simulink library "arsenal"  (R2025b)
settings: Solver=VariableStepAuto  StartTime=0.0  StopTime=10.0  RelTol=1e-3
undefined symbols (not defined in the file or in its folder): DiscIntNeverNeededParam, Kd
libraries: fl_lib x21, sdl_lib x4, simulink x3, dspstat3 x2, ee_lib x2, nesl_utility x2, simulink_extras x1, slpidlib x1
settings Model: Creator=upattacini  LastModifiedBy=upattacini

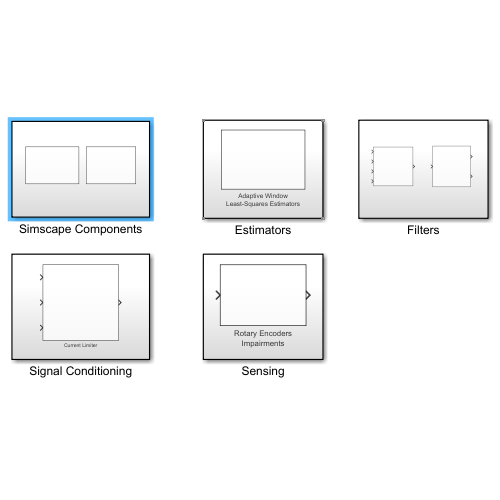
[thumbnail: Simulink's stored preview of the top-level diagram]
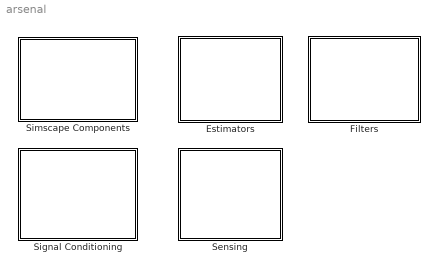
== system arsenal ==
  Estimators : Subsystem
  Filters : Subsystem
  Sensing : Subsystem
  Signal Conditioning : Subsystem
  Simscape Components : Subsystem

== system arsenal/Estimators ==
  Adaptive Window Least-Squares Estimators : Subsystem

== system arsenal/Filters ==
  Adaptive Exponential Smoother : Subsystem  mask(Exponential Adaptive Smoother){eta=0, m=0, V0=0}
      mask prompts: eta "Learning rate"; m "Momentum rate"; V0 "Initial variance estimate"
      mask help: Smooths out a noisy signal by estimating its variance at each time step. Use the learning rate to adjust the convergence speed and the momentum rate to weigh the noise applied to the gradient.
      mask Display:
      | port_label('input', 1, 'x','texmode', 'on');
      | port_label('output', 1, 'y','texmode', 'on');
      | port_label('output', 2, '\sigma^2_{est}','texmode', 'on');
  Discrete Minimum Jerk : Subsystem  mask(Minimum Jerk Filter){Ts=0.001}
      mask prompts: Ts "Sample time (s)"
      mask help:
      | Apply quasi-minimum jerk filtering to the input.
      | The filter reactivity can be adjusted via the input T, which specifies the rise-time.
      | The filter can be reset to output the initial value out0.

== system arsenal/Sensing ==
  Rotary Encoders Impairments : Subsystem  mask(Rotary Encoders Impairments){bit_resolution=14, bit_noise=2, seed=0, Ts=0.001}
      mask prompts: bit_resolution "Bits or resolution"; bit_noise "Bits of noise"; Ts "Sample time (s)"
      mask help:
      | Simulate the impairments underlying the rotary encoders readouts.
      | In particular, the block simulates the effects of quantization and noise.

== system arsenal/Signal Conditioning ==
  Current Limiter : Subsystem  mask(Current Limiter){Ts=0.00005, I_max_gain=0.1, Discrete_time_integrator_gain=1.0}
      mask prompts: Ts "Sample Time (s):"; I_max_gain "I Max Gain:"; Discrete_time_integrator_gain "Discrete-Time Integrator Gain:"
      mask help: This block limits the magnitude of an input current signal to a specified maximum value, preventing it from exceeding safe operating boundaries. It acts as a saturation filter to protect downstream components (such as motor drivers or actuators) from overcurrent conditions.
      mask TypeOptions Ts:
      | Discrete-Time
      | Integrator/SampleTime | Unit Delay/SampleTime
      mask TypeOptions I_max_gain: I_max_gain/Gain
      mask TypeOptions Discrete_time_integrator_gain:
      | Discrete-Time
      | Integrator/gainval

== system arsenal/Simscape Components ==
  Actuators : Subsystem
  Transmissions : Subsystem

== system arsenal/Estimators/Adaptive Window Least-Squares Estimators ==
  AWLS Estimator 1st-order : MATLAB Function  Description=This block implements adaptive window techniques as per https://dx.doi.org/10.1109/87.880606.  TreatAsAtomicUnit=on
  AWLS Estimator 2nd-order : MATLAB Function  Description=This block implements adaptive window techniques as per https://dx.doi.org/10.1109/87.880606.  TreatAsAtomicUnit=on

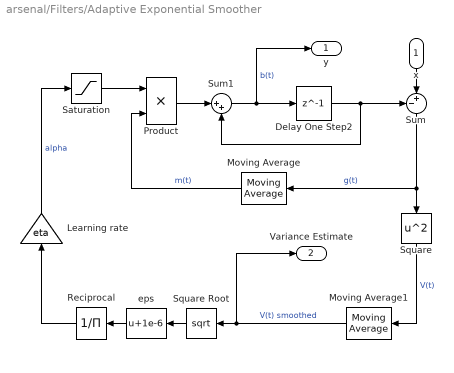
== system arsenal/Filters/Adaptive Exponential Smoother ==
  x : Inport  OutDataTypeStr=single
  Delay One Step2 : Delay  DelayLength=1  InitialCondition=0
  Learning rate : Gain  Gain=eta
  Moving Average : dspstat3/Moving Average  Method=Exponential weighting  ForgettingFactorPort=off  SpecifyWindowLength=on  WindowLength=4  OverlapLength=3  AllowArbitraryInputLength=off  ForgettingFactor=m  SimulateUsing=Code generation
  Moving Average1 : dspstat3/Moving Average  Method=Exponential weighting  ForgettingFactorPort=off  SpecifyWindowLength=on  WindowLength=4  OverlapLength=3  AllowArbitraryInputLength=off  ForgettingFactor=m  SimulateUsing=Code generation
  Product : Product
  Reciprocal : Product  Inputs=/  CollapseDim=2
  Saturation : Saturate  UpperLimit=0.99999  LowerLimit=1e-6
  Square : Math  Operator=square
  Square Root : Sqrt
  Sum : Sum  Inputs=-+|
  Sum1 : Sum  Inputs=|++
  eps : Bias  Bias=1e-6  SaturateOnIntegerOverflow=off
  y : Outport  OutDataTypeStr=single
  Variance Estimate : Outport  Port=2  VectorParamsAs1DForOutWhenUnconnected=off
  wires:
  Square Root/1 -> eps/1
  Sum/1 -> Moving Average/1, Square/1  "g(t)"
  eps/1 -> Reciprocal/1
  x/1 -> Sum/2
  Saturation/1 -> Product/1
  Reciprocal/1 -> Learning rate/1
  Learning rate/1 -> Saturation/1  "alpha"
  Product/1 -> Sum1/1
  Moving Average/1 -> Product/2  "m(t)"
  Moving Average1/1 -> Variance Estimate/1, Square Root/1  "V(t) smoothed"
  Square/1 -> Moving Average1/1  "V(t)"
  Sum1/1 -> Delay One Step2/1, y/1  "b(t)"
  Delay One Step2/1 -> Sum1/2, Sum/1

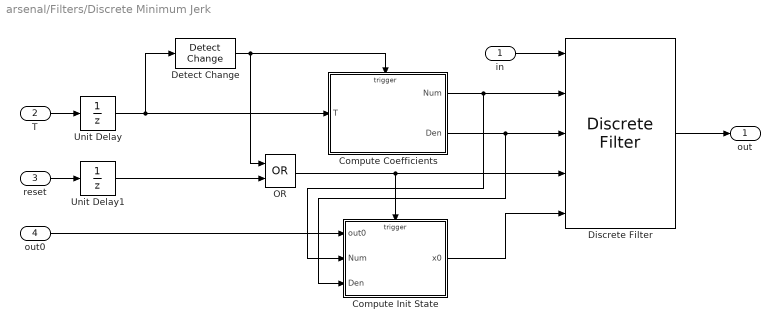
== system arsenal/Filters/Discrete Minimum Jerk ==
  in : Inport  PortDimensions=1
  T : Inport  Port=2  PortDimensions=1
  reset : Inport  Port=3  PortDimensions=1
  out0 : Inport  Port=4  PortDimensions=1
  Compute Coefficients : Subsystem
  Compute Init State : Subsystem  TreatAsAtomicUnit=on
  Detect Change : simulink/Logic and Bit Operations/Detect Change  vinit=0  OutDataTypeStr=uint8
  Discrete Filter : DiscreteFilter  NumeratorSource=Input port  DenominatorSource=Input port  InitialStatesSource=Input port  ExternalReset=Rising  a0EqualsOne=on
      settings: InputPortMap=u0,p1,p3,r7,p5
  OR : Logic  Operator=OR  AllPortsSameDT=off  OutDataTypeStr=boolean
  Unit Delay : UnitDelay  SampleTime=-1  HasFrameUpgradeWarning=on
  Unit Delay1 : UnitDelay  SampleTime=-1  HasFrameUpgradeWarning=on
  out : Outport  PortDimensions=1
  wires:
  in/1 -> Discrete Filter/1
  Discrete Filter/1 -> out/1
  T/1 -> Unit Delay/1
  Detect Change/1 -> Compute Coefficients/Trigger, OR/1
  Compute Coefficients/1(Num) -> Compute Init State/2(Num), Discrete Filter/2
  Compute Coefficients/2(Den) -> Compute Init State/3(Den), Discrete Filter/3
  Unit Delay/1 -> Compute Coefficients/1(T), Detect Change/1
  reset/1 -> Unit Delay1/1
  out0/1 -> Compute Init State/1(out0)
  Compute Init State/1(x0) -> Discrete Filter/5
  Unit Delay1/1 -> OR/2
  OR/1 -> Compute Init State/Trigger, Discrete Filter/4

== system arsenal/Sensing/Rotary Encoders Impairments ==
  in : Inport
  Quantization and Noise : Subsystem  mask{bit_resolution=bit_resolution, bit_noise=bit_noise, seed=0, Ts=Ts}
      mask prompts: bit_resolution "Resolution bits"; bit_noise "Noise bits"; Ts "Sample time (s)"
      settings: PortSchema="{\"entries\":[{\"content\":{\"sides\":[{\"content\":{\"connectorIds\":[\"Out1\"]},\"type\":\"ConnectorPlacement.EquallySpacedRectSide\",\"uuid\":\"5c60203e-1477-4c63-bf85-2a9264896243\"},{\"content\":{\"connectorIds\":[\"In1\"],\"side\":\"RIGHT\"},\"type\":\"ConnectorPlacement.EquallySpacedRectSide\",\"uuid\":\"fde9215e-0eee-4b90-b3d3-bc5e0578faf0\"},{\"content\":{\"side\":\"TOP\"},\"type\":\"ConnectorPlacement.EquallySpacedRectSide\",\"uuid\":\"75472767-9856-4b99-a0f4-bd856ef58e73\"}]},\"type\":\"ConnectorPlacement.EquallySpacedConnector\",\"uuid\":\"089ac2bf-9317-43ab-ab34-2d9e1bbbe948\"}],\"packageUris\":[\"http://schema.mathworks.com/mf0/Connector/R2020b\"],\"version\":\"1.0\"}"
  Signal Specification : SignalSpecification  Unit=deg
  Signal Specification1 : SignalSpecification  Unit=deg
  out : Outport
  wires:
  in/1 -> Signal Specification1/1
  Quantization and Noise/1(out) -> Signal Specification/1
  Signal Specification/1 -> out/1
  Signal Specification1/1 -> Quantization and Noise/1(in)

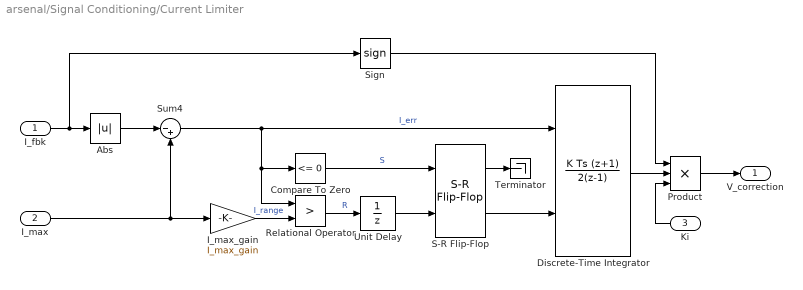
== system arsenal/Signal Conditioning/Current Limiter ==
  I_fbk : Inport
  I_max : Inport  Port=2
  Ki : Inport  Port=3
  Abs : Abs  ZeroCross=off  SaturateOnIntegerOverflow=off
  Compare To Zero : simulink/Logic and Bit Operations/Compare To Zero  relop=<=  OutDataTypeStr=boolean
  Discrete-Time Integrator : DiscreteIntegrator  IntegratorMethod=Integration: Trapezoidal  gainval=Discrete_time_integrator_gain  ExternalReset=level  SampleTime=Ts  ICPrevOutput=DiscIntNeverNeededParam  ICPrevScaledInput=DiscIntNeverNeededParam
  I_max_gain : Gain  Gain=I_max_gain  OutDataTypeStr=single
  Product : Product  Inputs=3
  Relational Operator : RelationalOperator  Operator=>  OutDataTypeStr=boolean  RndMeth=Simplest  InputSameDT=off
  S-R Flip-Flop : simulink_extras/Flip Flops/S-R Flip-Flop  initial_condition=0
  Sign : Signum
  Sum4 : Sum  Inputs=|-+
  Terminator : Terminator
  Unit Delay : UnitDelay  SampleTime=Ts  HasFrameUpgradeWarning=on
  V_correction : Outport
  wires:
  Discrete-Time Integrator/1 -> Product/2
  I_max_gain/1 -> Relational Operator/2  "I_range"
  S-R Flip-Flop/1 -> Terminator/1
  Abs/1 -> Sum4/1
  Sign/1 -> Product/1
  S-R Flip-Flop/2 -> Discrete-Time Integrator/2
  Sum4/1 -> Relational Operator/1, Compare To Zero/1, Discrete-Time Integrator/1  "I_err"
  Ki/1 -> Product/3
  I_fbk/1 -> Sign/1, Abs/1
  Compare To Zero/1 -> S-R Flip-Flop/1  "S"
  Relational Operator/1 -> Unit Delay/1  "R"
  I_max/1 -> Sum4/2, I_max_gain/1
  Product/1 -> V_correction/1
  Unit Delay/1 -> S-R Flip-Flop/2

== system arsenal/Simscape Components/Actuators ==
  DC Motors : Subsystem

== system arsenal/Simscape Components/Transmissions ==
  Harmonic Drives : Subsystem

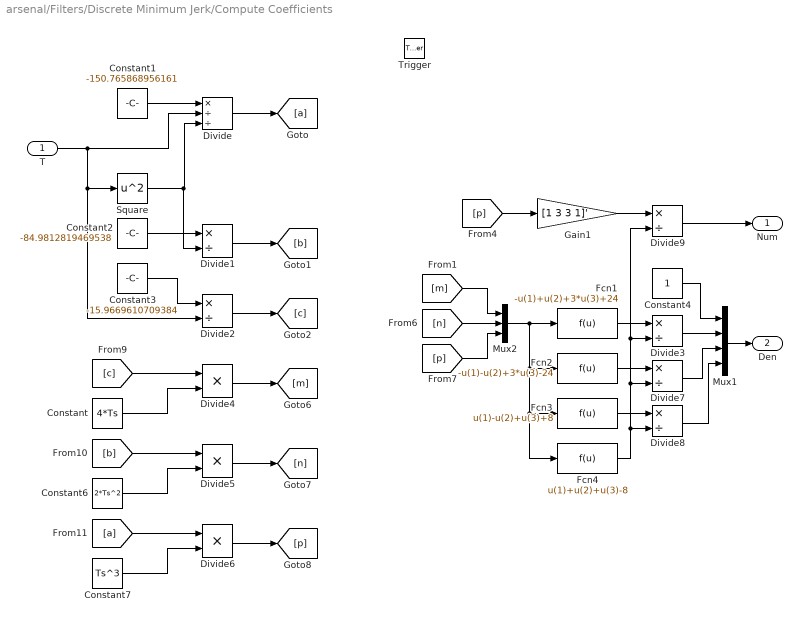
== system arsenal/Filters/Discrete Minimum Jerk/Compute Coefficients ==
  T : Inport
  Trigger : TriggerPort  VariantControl=(inherit)  PortDimensions=1
  Constant : Constant  Value=4*Ts
  Constant1 : Constant  Value=-150.765868956161
  Constant2 : Constant  Value=-84.9812819469538
  Constant3 : Constant  Value=-15.9669610709384
  Constant4 : Constant
  Constant6 : Constant  Value=2*Ts^2
  Constant7 : Constant  Value=Ts^3
  Divide : Product  Inputs=*//
  Divide{1..3,7..9} (6 alike) : Product  Inputs=*/
  Divide4 : Product  Inputs=**
  Divide5 : Product  Inputs=**
  Divide6 : Product  Inputs=**
  Fcn1 : Fcn  Expr=-u(1)+u(2)+3*u(3)+24
  Fcn2 : Fcn  Expr=-u(1)-u(2)+3*u(3)-24
  Fcn3 : Fcn  Expr=u(1)-u(2)+u(3)+8
  Fcn4 : Fcn  Expr=u(1)+u(2)+u(3)-8
  Gain1 : Gain  Gain=[1 3 3 1]'
  Mux1 : Mux
  Mux2 : Mux  Inputs=3
  Square : Math  Operator=square
  Num : Outport  InitialOutput=[0 0 0 0]
  Den : Outport  Port=2  InitialOutput=[1 0 0 0]'
  wires:
  Divide9/1 -> Num/1
  Gain1/1 -> Divide9/1
  Fcn4/1 -> Divide3/2, Divide9/2, Divide7/2, Divide8/2
  Fcn3/1 -> Divide8/1
  Fcn2/1 -> Divide7/1
  Divide8/1 -> Mux1/4
  Divide7/1 -> Mux1/3
  Divide3/1 -> Mux1/2
  Fcn1/1 -> Divide3/1
  Mux2/1 -> Fcn1/1, Fcn2/1, Fcn3/1, Fcn4/1
  [p] -> Mux2/3
  [n] -> Mux2/2
  [m] -> Mux2/1
  Constant7/1 -> Divide6/2
  [a] -> Divide6/1
  Divide6/1 -> [p]
  Divide5/1 -> [n]
  [b] -> Divide5/1
  Constant6/1 -> Divide5/2
  Constant/1 -> Divide4/2
  [c] -> Divide4/1
  Divide4/1 -> [m]
  Mux1/1 -> Den/1
  Constant4/1 -> Mux1/1
  Divide/1 -> [a]
  Square/1 -> Divide/3, Divide1/2
  Constant3/1 -> Divide2/1
  Constant2/1 -> Divide1/1
  [p] -> Gain1/1
  Divide2/1 -> [c]
  T/1 -> Divide/2, Square/1, Divide2/2
  Divide1/1 -> [b]
  Constant1/1 -> Divide/1

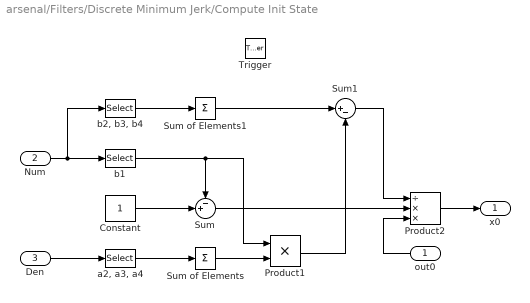
== system arsenal/Filters/Discrete Minimum Jerk/Compute Init State ==
  out0 : Inport
  Num : Inport  Port=2
  Den : Inport  Port=3
  Trigger : TriggerPort  VariantControl=(inherit)
  Constant : Constant
  Product1 : Product
  Product2 : Product  Inputs=/**
  Sum : Sum  Inputs=-+|
  Sum of Elements : Sum  Inputs=+
  Sum of Elements1 : Sum  Inputs=+
  Sum1 : Sum  Inputs=|+-
  "a2, a3, a4" : Selector  InputPortWidth=4  IndexOptions=Index vector (dialog)  Indices=[2 3 4]  OutputSizes=1
  b1 : Selector  InputPortWidth=4  IndexOptions=Index vector (dialog)  Indices=1  OutputSizes=1
  "b2, b3, b4" : Selector  InputPortWidth=4  IndexOptions=Index vector (dialog)  Indices=[2 3 4]  OutputSizes=1
  x0 : Outport
  wires:
  Den/1 -> "a2, a3, a4"/1
  Num/1 -> "b2, b3, b4"/1, b1/1
  Constant/1 -> Sum/2
  b1/1 -> Sum/1, Product1/1
  "a2, a3, a4"/1 -> Sum of Elements/1
  "b2, b3, b4"/1 -> Sum of Elements1/1
  Sum of Elements/1 -> Product1/2
  Sum of Elements1/1 -> Sum1/1
  Product1/1 -> Sum1/2
  Sum/1 -> Product2/2
  Sum1/1 -> Product2/1
  out0/1 -> Product2/3
  Product2/1 -> x0/1

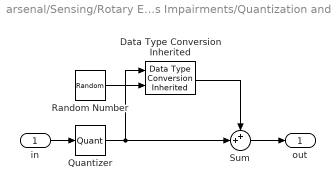
== system arsenal/Sensing/Rotary Encoders Impairments/Quantization and Noise ==
  in : Inport
  Data Type Conversion Inherited : simulink/Signal Attributes/Data Type Conversion Inherited  ConvertRealWorld=Real World Value  DoSatur=off
  Quantizer : Quantizer  QuantizationInterval=360/2^bit_resolution
  Random Number : RandomNumber  Variance=((360/2^bit_resolution)*(2^bit_noise-1) * (1/3))^2  Seed=seed  SampleTime=Ts
  Sum : Sum  Inputs=++|
  out : Outport
  wires:
  Quantizer/1 -> Data Type Conversion Inherited/1, Sum/2
  Random Number/1 -> Data Type Conversion Inherited/2
  in/1 -> Quantizer/1
  Sum/1 -> out/1
  Data Type Conversion Inherited/1 -> Sum/1

== system arsenal/Simscape Components/Actuators/DC Motors ==
  DC Motor Drive : Subsystem  mask{R=0.58, L=0.0002, Kt=0.1564, T_bkpts=[0 0.774 1.564 2.71], I_table=[0 4.95 10 17.325], V_rated=48, GB_ratio=7.75, J=6.9927e-5, Kp=0.1, Ki=0.1, Ts=0.005, ff_bkpts=[0 60 120 180 240 310], ff_table=[0 10 20 40 60 80], V_max=100}
      mask prompts: R "Armature Resistance (Ohm)"; L "Armataure Inductabce (H)"; Kt "Torque Constant (Nm/A)"; T_bkpts "Torque breakpoints (Nm)"; I_table "Current table (A)"; V_rated "Rated DC Voltage (V)"; GB_ratio "Gearbox Ratio"; J "Rotor Inertia (kgm^2)"; Kp "Speed Controller Kp (1/rpm)"; Ki "Speed Controller Ki (1/(rpm*s))"; Ts "Speed Controller Sample Time (s)"; ff_bkpts "Speed Controller FF breakpoints (rpm)"; ff_table "Speed Controller FF table (%)"; V_max "Speed Controller Max Voltage (%)"
      mask init:
      | p = polyfit(T_bkpts, I_table, 1);
      |     I_noload = max([p(2) 0]);
      |     clear p;
      mask Display:
      | % Circle
      | plot(sin(0:0.1:2.2*pi)*0.9,cos(0:0.1:2.2*pi)*0.9);
      | 
      | % In/out
      | plot([-1.1 -0.9],[0 0]);
      | plot([1.1 0.9],[0 0]);
      | 
      | % 'M'
      | plot([0.5 0.5],[-0.5 0.5]);
      | plot([-0.5 -0.5],[-0.5 0.5]);
      | plot([0.5 0],[0.5 -0.5]);
      | plot([-0.5 0],[0.5 -0.5]);
      | 
      | % Plot points to set plot range
      | color('white');plot(1.9,1.2);plot(-1.9,-1.2)
      | color('black');
      | 
      | port_label('input', 1, 'w_ref');
      | port_label('lconn', 1, 'V');
      | 
      | port_label('output', 1, 'DC');
      | port_label('rconn', 1, 'R');
      | port_label('rconn', 2, 'w');
      | port_label('rconn', 3, 'I');
      | port_label('rconn', 4, 'T');
      | port_label('rconn', 5, 'P');

== system arsenal/Simscape Components/Transmissions/Harmonic Drives ==
  HFUC_8_2A : Subsystem

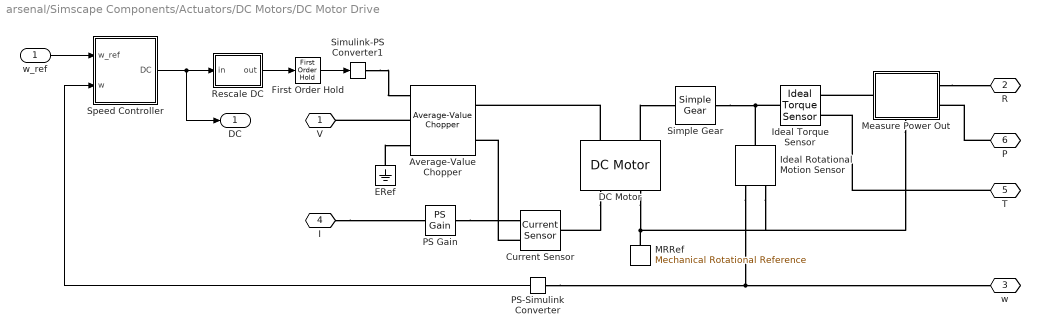
== system arsenal/Simscape Components/Actuators/DC Motors/DC Motor Drive ==
  w_ref : Inport  Unit=rpm
  Average-Value Chopper : ee_lib/Semiconductors & Converters/Converters/Average-Value Chopper  chopper_type=5  efficiency_option=1  efficiency_fixed=100  i_vec=[0, 2, 5] A  efficiency_vec=[90, 95, 98]
      settings: InternalSimscapePortConfiguration="{\"Bottom\":[],\"Left\":[{\"id\":\"DutyCycle\",\"label\":\"DutyCycle\",\"type\":\"input\"},{\"id\":\"p1\",\"label\":\"1+\",\"type\":\"foundation.electrical.electrical\"},{\"id\":\"n1\",\"label\":\"1-\",\"type\":\"foundation.electrical.electrical\"}],\"Right\":[{\"id\":\"p2\",\"label\":\"2+\",\"type\":\"foundation.electrical.electrical\"},{\"id\":\"n2\",\"label\":\"2-\",\"type\":\"foundation.electrical.electrical\"}],\"Top\":[]}"
  Current Sensor : fl_lib/Electrical/Electrical Sensors/Current Sensor
  DC Motor : ee_lib/Electromechanical/Brushed Motors/DC Motor  field_option=ee.enum.field_option.pm  Rf=100 Ohm  Lf=1 H  Laf=0.15 H  If0=0 A  parameterization=ee.enum.dcparam_option.circuit_param  Ra=R Ohm  La=L H  emf_or_torque=ee.enum.emf_or_torque.ki  Kv=4.7 / 1000 V/rpm  Ki=Kt N*m/A  T_stall=T_stall N*m  w_max=vel_noload rpm  w_rated="vel_rated  rpm"  P_rated=P_rated W  V_rated=V_rated V  lam_param=ee.enum.lam_param.current  i_noload=I_noload A  V_i_noload=V_rated V  J=J kg*m^2  lam=0 N*m*s/rad  speed0=0 rpm  alpha=3.93e-3 1/K  Tmeas=25 degC  thermal_mass=100 J/K  initial_temperature=25 degC
  ERef : fl_lib/Electrical/Electrical Elements/Electrical Reference
  First Order Hold : FirstOrderHold  InitialOutput=0.5  ErrorTolerance=inf
  Ideal Rotational Motion Sensor : fl_lib/Mechanical/Mechanical Sensors/Ideal Rotational Motion Sensor  reference=foundation.enum.MeasurementReference.difference  acceleration_port=false  velocity_port=true  position_port=false  wrap_angle=false  offset=0 rad
      settings: InternalSimscapePortConfiguration="{\"Bottom\":[],\"Left\":[{\"id\":\"R\",\"label\":\"R\",\"type\":\"foundation.mechanical.rotational.rotational\"}],\"Right\":[{\"id\":\"C\",\"label\":\"C\",\"type\":\"foundation.mechanical.rotational.rotational\"},{\"id\":\"W\",\"label\":\"W\",\"type\":\"output\"}],\"Top\":[]}"
  Ideal Torque Sensor : fl_lib/Mechanical/Mechanical Sensors/Ideal Torque Sensor
  MRRef : fl_lib/Mechanical/Rotational Elements/Mechanical Rotational Reference
  Measure Power Out : Subsystem
      settings: PortSchema="{\"entries\":[{\"content\":{\"sides\":[{\"content\":{\"connectorIds\":[\"LConn1\"]},\"type\":\"ConnectorPlacement.EquallySpacedRectSide\",\"uuid\":\"ab2aa2ce-2cbf-45e7-81ae-2c0fe77a52cc\"},{\"content\":{\"connectorIds\":[\"RConn1\",\"RConn2\"],\"side\":\"RIGHT\"},\"type\":\"ConnectorPlacement.EquallySpacedRectSide\",\"uuid\":\"5c982c99-0472-49ff-a868-bdbf2d84961a\"},{\"content\":{\"side\":\"TOP\"},\"type\":\"ConnectorPlacement.EquallySpacedRectSide\",\"uuid\":\"0e0fcf9a-da83-4384-8a48-478a089b4976\"},{\"content\":{\"connectorIds\":[\"RConn3\"],\"side\":\"BOTTOM\"},\"type\":\"ConnectorPlacement.EquallySpacedRectSide\",\"uuid\":\"0e4cf7cc-8767-4594-ba20-9b51fc69446f\"}]},\"type\":\"ConnectorPlacement.EquallySpacedConnector\",\"uuid\":\"1ebf3542-a9ec-43c2-821e-3013d7d98f30\"}],\"packageUris\":[\"http://schema.mathworks.com/mf0/Connector/R2020b\"],\"version\":\"1.0\"}"
      mask Display: disp('P');
  PS Gain : fl_lib/Physical Signals/Functions/PS Gain  gain=1 / sqrt(3/2)
  PS-Simulink Converter : nesl_utility/PS-Simulink Converter  PhysicalDomain=network_engine_domain  SubClassName=ps_output  LeftPortType=input  RightPortType=output  PseudoPeriodic=off  Frequencies=[]  VectorFormat=inherit  Unit=rpm  AffineConversion=off
  Rescale DC : Subsystem
      mask Display: disp('Rescale');
  Simple Gear : sdl_lib/Gears/Simple Gear  ratio=GB_ratio  rotation_direction=sdl.enum.shaftOutputDirection.same  friction_model=sdl.enum.gear_efficiencies_load.off  T_noload=0.1 N*m  T_nom=5 N*m  efficiency_nom=0.8  efficiency=0.8  temperature_TLU=[280, 300, 320] K  load_TLU=[1, 5, 10] N*m  efficiency_TLU=[.95, .9, .85]  efficiency_TLU2=[.85, .8, .75; .95, .9, .85; .85, .8, .7]  w_thr=0.01 rad/s  pwr_thr=0.001 W  enable_backlash=false  hardstop_model=simscape.enum.hardstop.smooth  backlash_distance=1e-3 mm  r_base=0.1 m  transition=1e-4 mm  backlash_stiffness=1e6 N/m  backlash_damping=1e3 N*s/m  coeff_rest=0.7  v_tol=0.001 m/s  f_tol=0.001 N  mu_visc=[0, 0] N*m*s/rad  thermal_mass=50 J/K  temperature_specify=off  temperature_priority=High  temperature=300 K  temperature_nominal_specify=off  temperature_nominal_value=1  temperature_nominal_unit=K  x_backlash_specify=off  x_backlash_priority=None  x_backlash=0 mm  x_backlash_nominal_specify=off  x_backlash_nominal_value=1  x_backlash_nominal_unit=mm  f_hardstop_specify=off  f_hardstop_priority=None  f_hardstop=0 N  f_hardstop_nominal_specify=off  f_hardstop_nominal_value=1  f_hardstop_nominal_unit=N  v_backlash_specify=off  v_backlash_priority=None  v_backlash=0 m/s  v_backlash_nominal_specify=off  v_backlash_nominal_value=1  v_backlash_nominal_unit=m/s
  Simulink-PS Converter1 : nesl_utility/Simulink-PS Converter  PhysicalDomain=network_engine_domain  SubClassName=ps_input  LeftPortType=input  RightPortType=output  PseudoPeriodic=off  Frequencies=[]  NoiseDistribution=none  NoiseParameters=[]  Unit=1  AffineConversion=off  FilteringAndDerivatives=filter  SimscapeFilterOrder=1  InputFilterTimeConstant=Ts/10  UdotUserProvided=0
  Speed Controller : Subsystem
  V : PMIOPort  Side=Left
  R : PMIOPort  Port=2  Side=Right
  w : PMIOPort  Port=3  Side=Right
  I : PMIOPort  Port=4  Side=Right
  T : PMIOPort  Port=5  Side=Right
  P : PMIOPort  Port=6  Side=Right
  DC : Outport  Unit=%
  wires:
  PS-Simulink Converter/1 -> Speed Controller/2(w)
  First Order Hold/1 -> Simulink-PS Converter1/1
  Speed Controller/1(DC) -> Rescale DC/1(in), DC/1
  w_ref/1 -> Speed Controller/1(w_ref)
  Rescale DC/1(out) -> First Order Hold/1
  connections:
  MRRef/LConn1 -- DC Motor/RConn2 -- Ideal Rotational Motion Sensor/RConn1 -- Measure Power Out/RConn3
  Ideal Rotational Motion Sensor/RConn2 -- w/RConn1 -- PS-Simulink Converter/LConn1
  Ideal Rotational Motion Sensor/LConn1 -- Simple Gear/RConn1 -- Ideal Torque Sensor/LConn1
  T/RConn1 -- Ideal Torque Sensor/RConn2
  ERef/LConn1 -- Average-Value Chopper/LConn3
  PS Gain/LConn1 -- Current Sensor/RConn1
  P/RConn1 -- Measure Power Out/RConn2
  Measure Power Out/RConn1 -- R/RConn1
  Current Sensor/RConn2 -- Average-Value Chopper/RConn2
  Simulink-PS Converter1/RConn1 -- Average-Value Chopper/LConn1
  I/RConn1 -- PS Gain/RConn1
  DC Motor/LConn1 -- Average-Value Chopper/RConn1
  Average-Value Chopper/LConn2 -- V/RConn1
  Measure Power Out/LConn1 -- Ideal Torque Sensor/RConn1
  DC Motor/RConn1 -- Current Sensor/LConn1
  DC Motor/LConn2 -- Simple Gear/LConn1

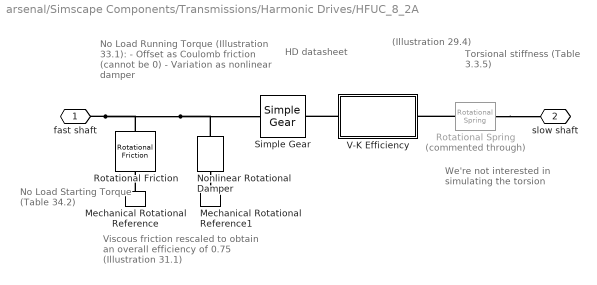
== system arsenal/Simscape Components/Transmissions/Harmonic Drives/HFUC_8_2A ==
  note: No Load Starting Torque
      | (Table 34.2)
  note: No Load Running Torque (Illustration 33.1):
      | - Offset as Coulomb friction (cannot be 0)
      | - Variation as nonlinear damper
  note: Torsional stiffness
      | (Table 3.3.5)
  note: Viscous friction rescaled to obtain an
      | overall efficiency of 0.75 (Illustration 31.1)
  note: (Illustration 29.4)
  note: HD datasheet
  note: We're not interested in
      | simulating the torsion
  Mechanical Rotational Reference : fl_lib/Mechanical/Rotational Elements/Mechanical Rotational Reference
  Mechanical Rotational Reference1 : fl_lib/Mechanical/Rotational Elements/Mechanical Rotational Reference
  Nonlinear Rotational Damper : sdl_lib/Couplings & Drives/Springs & Dampers/Nonlinear Rotational Damper  parameterization=sdl.enum.polynomialTLU.tlu  symmetry=sdl.enum.symmetry.symmetric  coefficient_vector=[.0001, 0, 1e-05, 0, 1e-06] N*m*s/rad  positive_coefficient_vector=[.0001, 0, 1e-05, 0, 1e-06] N*m*s/rad  negative_coefficient_vector=[.001, -1e-05, .0001, 0, 0] N*m*s/rad  angular_velocity_vector=[-3500, -2000, -1000, -500, 500, 1000, 2000, 3500] rpm  torque_vector=[-0.7, -0.2, -0.1, 0, 0, 0.1, 0.2, 0.7]*0.5 N*cm  interp_method=simscape.enum.interpolation.linear  extrap_method=simscape.enum.extrapolation.nearest
      settings: InternalSimscapePortConfiguration="{\"Bottom\":[],\"Left\":[{\"id\":\"R\",\"label\":\"R\",\"type\":\"foundation.mechanical.rotational.rotational\"}],\"Right\":[{\"id\":\"C\",\"label\":\"C\",\"type\":\"foundation.mechanical.rotational.rotational\"}],\"Top\":[]}"
  Rotational Friction : fl_lib/Mechanical/Rotational Elements/Rotational Friction  brkwy_trq=0.59 N*cm  brkwy_vel=0.001 rad/s  Col_trq=0.3*0.5 N*cm  visc_coef=0 N*cm/rpm  w_specify=off  w_priority=None  w=0 rad/s  w_nominal_specify=off  w_nominal_value=1  w_nominal_unit=rad/s  t_specify=off  t_priority=None  t=0 N*m  t_nominal_specify=off  t_nominal_value=1  t_nominal_unit=N*m
  Rotational Spring : fl_lib/Mechanical/Rotational Elements/Rotational Spring  Commented=through  spr_rate=1000 N*m/rad  w_specify=off  w_priority=None  w=0 rad/s  w_nominal_specify=off  w_nominal_value=1  w_nominal_unit=rad/s  t_specify=off  t_priority=None  t=0 N*m  t_nominal_specify=off  t_nominal_value=1  t_nominal_unit=N*m  phi_specify=off  phi_priority=High  phi=0 rad  phi_nominal_specify=off  phi_nominal_value=1  phi_nominal_unit=rad
  Simple Gear : sdl_lib/Gears/Simple Gear  ratio=100  rotation_direction=sdl.enum.shaftOutputDirection.opposite  friction_model=sdl.enum.gear_efficiencies_load.off  T_noload=0.1 N*m  T_nom=5 N*m  efficiency_nom=0.8  efficiency=1  temperature_TLU=[280, 300, 320] K  load_TLU=[1, 5, 10] N*m  efficiency_TLU=[.95, .9, .85]  efficiency_TLU2=[.85, .8, .75; .95, .9, .85; .85, .8, .7]  w_thr=0.01 rad/s  pwr_thr=0.001 W  enable_backlash=false  hardstop_model=simscape.enum.hardstop.smooth  backlash_distance=1e-3 mm  r_base=0.1 m  transition=1e-4 mm  backlash_stiffness=1e6 N/m  backlash_damping=1e3 N*s/m  coeff_rest=0.7  v_tol=0.001 m/s  f_tol=0.001 N  mu_visc=[0, 0] N*cm*s/rad  thermal_mass=50 J/K  temperature_specify=off  temperature_priority=High  temperature=300 K  temperature_nominal_specify=off  temperature_nominal_value=1  temperature_nominal_unit=K  x_backlash_specify=off  x_backlash_priority=None  x_backlash=0 mm  x_backlash_nominal_specify=off  x_backlash_nominal_value=1  x_backlash_nominal_unit=mm  f_hardstop_specify=off  f_hardstop_priority=None  f_hardstop=0 N  f_hardstop_nominal_specify=off  f_hardstop_nominal_value=1  f_hardstop_nominal_unit=N  v_backlash_specify=off  v_backlash_priority=None  v_backlash=0 m/s  v_backlash_nominal_specify=off  v_backlash_nominal_value=1  v_backlash_nominal_unit=m/s
  V-K Efficiency : Subsystem
  fast shaft : PMIOPort  Side=Left  ConnectionType=Connection: foundation.mechanical.rotational.rotational
  slow shaft : PMIOPort  Port=2  Side=Right  ConnectionType=Connection: foundation.mechanical.rotational.rotational
  connections:
  V-K Efficiency/LConn1 -- Simple Gear/RConn1
  Rotational Spring/LConn1 -- V-K Efficiency/RConn1
  Rotational Spring/RConn1 -- slow shaft/RConn1
  Nonlinear Rotational Damper/RConn1 -- Mechanical Rotational Reference1/LConn1
  Mechanical Rotational Reference/LConn1 -- Rotational Friction/RConn1
  fast shaft/RConn1 -- Rotational Friction/LConn1 -- Nonlinear Rotational Damper/LConn1 -- Simple Gear/LConn1

== system arsenal/Simscape Components/Actuators/DC Motors/DC Motor Drive/Measure Power Out ==
  Rotational Power Sensor : sdl_lib/Sensors/Rotational Power Sensor  measurement_type=sdl.enum.rotationalPowerSensorType.instantaneous  averaging_period=1 s  max_frequency=1000 Hz  max_speed=1000 rpm
      settings: InternalSimscapePortConfiguration="{\"Bottom\":[],\"Left\":[{\"id\":\"S\",\"label\":\"S\",\"type\":\"foundation.mechanical.rotational.rotational\"},{\"id\":\"R\",\"label\":\"R\",\"type\":\"foundation.mechanical.rotational.rotational\"},{\"id\":\"C\",\"label\":\"C\",\"type\":\"foundation.mechanical.rotational.rotational\"}],\"Right\":[{\"id\":\"P\",\"label\":\"P\",\"type\":\"output\"}],\"Top\":[]}"
  Conn1 : PMIOPort  Side=Left
  Conn2 : PMIOPort  Port=2  Side=Right
  P : PMIOPort  Port=3  Side=Right
  Conn3 : PMIOPort  Port=4  Side=Right
  connections:
  P/RConn1 -- Rotational Power Sensor/RConn1
  Conn1/RConn1 -- Rotational Power Sensor/LConn1
  Rotational Power Sensor/LConn2 -- Conn2/RConn1
  Conn3/RConn1 -- Rotational Power Sensor/LConn3

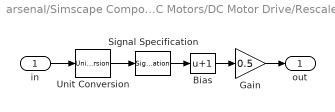
== system arsenal/Simscape Components/Actuators/DC Motors/DC Motor Drive/Rescale DC ==
  in : Inport
  Bias : Bias  Bias=1  SaturateOnIntegerOverflow=off
  Gain : Gain  Gain=0.5
  Signal Specification : SignalSpecification  Unit=1
  Unit Conversion : UnitConversion
  out : Outport
  wires:
  in/1 -> Unit Conversion/1
  Unit Conversion/1 -> Signal Specification/1
  Signal Specification/1 -> Bias/1
  Bias/1 -> Gain/1
  Gain/1 -> out/1

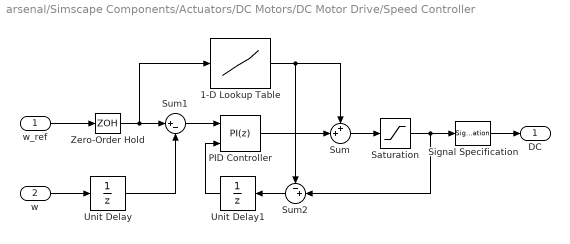
== system arsenal/Simscape Components/Actuators/DC Motors/DC Motor Drive/Speed Controller ==
  w_ref : Inport
  w : Inport  Port=2
  1-D Lookup Table : Lookup_n-D  NumberOfTableDimensions=1  BreakpointsForDimension1=[-fliplr(ff_bkpts(2:end)) ff_bkpts]  Table=[-fliplr(ff_table(2:end)) ff_table]  ExtrapMethod=Clip  InternalRulePriority=Speed  RndMeth=Simplest
  PID Controller : slpidlib/PID Controller  Controller=PI  Form=Parallel  TimeDomain=Discrete-time  UseExternalTs=off  SampleTime=Ts  IntegratorMethod=Trapezoidal  FilterMethod=Trapezoidal  ControllerParametersSource=internal  P=Kp  I=Ki  UseKiTs=off  D=Kd  UseExternalDerivativeSource=off  N=100  UseFilter=on  TunerSelectOption=Transfer Function Based (PID Tuner App)  ZeroCross=off  InitialConditionSource=internal  InitialConditionForIntegrator=0  InitialConditionForFilter=0  DifferentiatorICPrevScaledInput=0  ExternalReset=none  TrackingMode=on  Kt=1  LimitOutput=off  SatLimitsSource=internal  UpperSaturationLimit=abs(V_max)  LowerSaturationLimit=-abs(V_max)  LinearizeAsGain=on  AntiWindupMode=clamping  Kb=1  LimitIntegrator=off  UpperIntegratorSaturationLimit=abs(V_max)  LowerIntegratorSaturationLimit=-abs(V_max)  POutMin=[]  POutMax=[]  IOutMin=[]  IOutMax=[]  DOutMin=[]  DOutMax=[]  NOutMin=[]  NOutMax=[]  SumOutMin=[]  SumOutMax=[]  SaturationOutMin=[]  SaturationOutMax=[]  PParamMin=[]  PParamMax=[]  IParamMin=[]  IParamMax=[]  DParamMin=[]  DParamMax=[]  NParamMin=[]  NParamMax=[]  KbParamMin=[]  KbParamMax=[]  KtParamMin=[]  KtParamMax=[]  KbOutMin=[]  KbOutMax=[]  KtOutMin=[]  KtOutMax=[]  IntegratorOutMin=[]  IntegratorOutMax=[]  FilterOutMin=[]  FilterOutMax=[]  SumI1OutMin=[]  SumI1OutMax=[]  SumI2OutMin=[]  SumI2OutMax=[]  SumI3OutMin=[]  SumI3OutMax=[]  SumI4OutMin=[]  SumI4OutMax=[]  SumDOutMin=[]  SumDOutMax=[]  DifferentiatorOutMin=[]  DifferentiatorOutMax=[]  FilterDiffOutCoefMin=[]  FilterDiffOutCoefMax=[]  ReciprocalOutMin=[]  ReciprocalOutMax=[]  SumDenOutMin=[]  SumDenOutMax=[]  SumNumOutMin=[]  SumNumOutMax=[]  DivideOutMin=[]  DivideOutMax=[]  UdiffTsProdOutMin=[]  UdiffTsProdOutMax=[]  NTsProdOutMin=[]  NTsProdOutMax=[]  UintegralTsProdOutMin=[]  UintegralTsProdOutMax=[]  UngainTsProdOutMin=[]  UngainTsProdOutMax=[]  ClampingZeroOutDataTypeStr=Inherit: Inherit via back propagation  ClampingZeroOutMin=[]  ClampingZeroOutMax=[]  FilterDenConstantOutDataTypeStr=Inherit: Inherit via back propagation  FilterDenConstantOutMin=[]  FilterDenConstantOutMax=[]  PCopyOutDataTypeStr=Inherit: Inherit via back propagation  PCopyOutMin=[]  PCopyOutMax=[]  NCopyOutDataTypeStr=Inherit: Inherit via back propagation  NCopyOutMin=[]  NCopyOutMax=[]  IntegratorContinuousStateAttributes=''  IntegratorStateMustResolveToSignalObject=off  IntegratorRTWStateStorageClass=Auto  FilterContinuousStateAttributes=''  FilterStateMustResolveToSignalObject=off  FilterRTWStateStorageClass=Auto  ParallelPVariant=InternalParameters  IdealPVariant=Disabled  IVariant=InternalParameters  DVariant=Disabled  IntegratorVariant=Discrete  SatVariant=Disabled  AWVariant=Passthrough  PCopyVariant=Disabled  TRVariant=Enabled  FdbkBlocksVariant=Feedback  IdealPFdbkVariant=Passthrough  SatFdbkVariant=Passthrough  DerivativeFilterVariant=Disabled  NVariant=Disabled  NCopyVariant=Disabled_SignalSpec  FilterICVariant=Disabled  IntegratorICVariant=InternalICs  ExternalResetVariant=Disabled  TRSumVariant=TrackingMode  SumFdbkVariant=Enabled  SumVariant=Sum_PI  TsampFilterVariant=InternalTs  TsampNgainVariant=Passthrough  TsampIntegralVariant=Disabled_SignalSpec  ExternalSaturationOutDataTypeStr=Inherit: Same as second input  DerivativeSourceVariant=Disabled  PreIntVariant=InternalPreInt
  Saturation : Saturate  UpperLimit=abs(V_max)  LowerLimit=-abs(V_max)
  Signal Specification : SignalSpecification  Unit=%
  Sum : Sum  Inputs=++|
  Sum1 : Sum  Inputs=|+-
  Sum2 : Sum  Inputs=-+|
  Unit Delay : UnitDelay  SampleTime=Ts  HasFrameUpgradeWarning=on
  Unit Delay1 : UnitDelay  SampleTime=Ts  HasFrameUpgradeWarning=on
  Zero-Order Hold : ZeroOrderHold  SampleTime=Ts
  DC : Outport
  wires:
  w_ref/1 -> Zero-Order Hold/1
  Signal Specification/1 -> DC/1
  Sum1/1 -> PID Controller/1
  Unit Delay/1 -> Sum1/2
  Zero-Order Hold/1 -> 1-D Lookup Table/1, Sum1/1
  w/1 -> Unit Delay/1
  Saturation/1 -> Sum2/2, Signal Specification/1
  Sum/1 -> Saturation/1
  PID Controller/1 -> Sum/2
  Sum2/1 -> Unit Delay1/1
  Unit Delay1/1 -> PID Controller/2
  1-D Lookup Table/1 -> Sum2/1, Sum/1

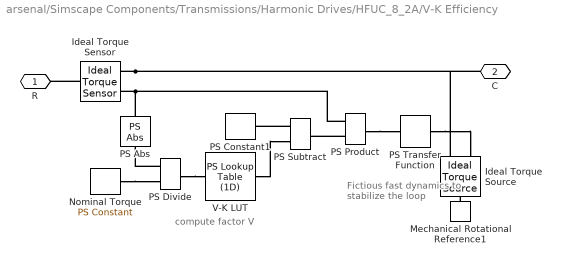
== system arsenal/Simscape Components/Transmissions/Harmonic Drives/HFUC_8_2A/V-K Efficiency ==
  note: Fictious fast dynamics
      | to stabilize the loop
  note: compute
      | factor V
  Ideal Torque Sensor : fl_lib/Mechanical/Mechanical Sensors/Ideal Torque Sensor
  Ideal Torque Source : fl_lib/Mechanical/Mechanical Sources/Ideal Torque Source
  Mechanical Rotational Reference1 : fl_lib/Mechanical/Rotational Elements/Mechanical Rotational Reference
  Nominal Torque : fl_lib/Physical Signals/Sources/PS Constant  constant=2.4 N*m
  PS Abs : fl_lib/Physical Signals/Nonlinear Operators/PS Abs  ZeroCross=true
      settings: InternalSimscapePortConfiguration="{\"Bottom\":[],\"Left\":[{\"id\":\"I\",\"label\":\"\",\"type\":\"input\"}],\"Right\":[{\"id\":\"O\",\"label\":\"\",\"type\":\"output\"}],\"Top\":[]}"
  PS Constant1 : fl_lib/Physical Signals/Sources/PS Constant  constant=1
  PS Divide : fl_lib/Physical Signals/Functions/PS Divide
  PS Product : fl_lib/Physical Signals/Functions/PS Product
  PS Subtract : fl_lib/Physical Signals/Functions/PS Subtract
  PS Transfer Function : fl_lib/Physical Signals/Linear Operators/PS Transfer Function  transfer_function_type=foundation.enum.transfer_function_type.lag  T=1e-6 s  T1=2 s  T2=1 s  reset_method=foundation.enum.IntegratorResetSpec.None  initial_condition_spec=foundation.enum.IntegratorICSpec.Internal  y0=0 N*m
      settings: InternalSimscapePortConfiguration="{\"Bottom\":[],\"Left\":[{\"id\":\"U\",\"label\":\"\",\"type\":\"input\"}],\"Right\":[{\"id\":\"Y\",\"label\":\"\",\"type\":\"output\"}],\"Top\":[]}"
  V-K LUT : fl_lib/Physical Signals/Lookup Tables/PS Lookup Table (1D)  x=[0.1, 0.2, 0.4, 0.6, 0.8, 1]  f=[0.45, 0.65, 0.85, 0.95, 0.99, 1]  interp_method=simscape.enum.interpolation.linear  extrap_method=simscape.enum.extrapolation.nearest
  R : PMIOPort  Side=Left
  C : PMIOPort  Port=2  Side=Right
  connections:
  PS Transfer Function/RConn1 -- Ideal Torque Source/RConn1
  Mechanical Rotational Reference1/LConn1 -- Ideal Torque Source/LConn1
  PS Product/RConn1 -- PS Transfer Function/LConn1
  PS Product/LConn2 -- PS Subtract/RConn1
  V-K LUT/RConn1 -- PS Subtract/LConn2
  PS Subtract/LConn1 -- PS Constant1/RConn1
  PS Divide/RConn1 -- V-K LUT/LConn1
  Nominal Torque/RConn1 -- PS Divide/LConn2
  Ideal Torque Sensor/RConn1 -- Ideal Torque Source/RConn2 -- C/RConn1
  Ideal Torque Sensor/LConn1 -- R/RConn1
  Ideal Torque Sensor/RConn2 -- PS Product/LConn1 -- PS Abs/LConn1
  PS Divide/LConn1 -- PS Abs/RConn1

== matlab function arsenal/Estimators/Adaptive Window Least-Squares Estimators/AWLS Estimator 1st-order ==
  data: y input; out output; d input; T input; N output
function [out,N]=awls1(y,d,T)
%#ok<*NASGU>

coder.extrinsic('polyfitHelper');

persistent n;
if isempty(n)
    n=1;
end

L=length(y);
pos=zeros(1,2);
Ly=0;
N=n;

for j=max(1,n-1):min(n+1,L-1)
    pos=polyfitHelper(y,1,T,j);

    finish=false;
    for i=0:j
        Ly=polyval(pos,i*T);
        if abs(y(L-j+i)-Ly)>d
            finish=true;
            break;
        end
    end
    
    if finish
        N=j;
        break;
    end
    N=j;
end

out=pos(1);
n=N;

== matlab function arsenal/Estimators/Adaptive Window Least-Squares Estimators/AWLS Estimator 2nd-order ==
  data: y input; out output; d input; T input; N output
function [out,N]=awls2(y,d,T)
%#ok<*NASGU>

coder.extrinsic('polyfitHelper');

persistent n;
if isempty(n)
    n=1;
end

L=length(y);
pos=zeros(1,3);
v=0;                
a=0;
Ly=0;
N=n;

for j=max(2,n-1):min(n+1,L-1)    
    pos=polyfitHelper(y,2,T,j);

    finish=false;
    for i=0:j
        Ly=polyval(pos,i*T);
        if abs(y(L-j+i)-Ly)>d
            finish=true;
            break;
        end
    end
    
    if finish
        N=j;
        break;
    end
    N=j;
end

out=2*pos(1);
n=N;
